simulink model "ACTIVITY_01_DR_CHAIREZ"  (R2022a)
settings: Solver=VariableStepAuto  StartTime=0.0  StopTime=1  RelTol=1e-3
libraries: slpidlib x2
settings Model: Creator=Pitip  LastModifiedBy=Pitip

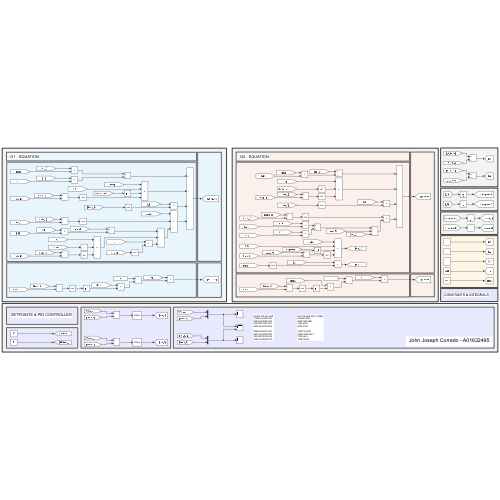
[thumbnail: Simulink's stored preview of the top-level diagram]
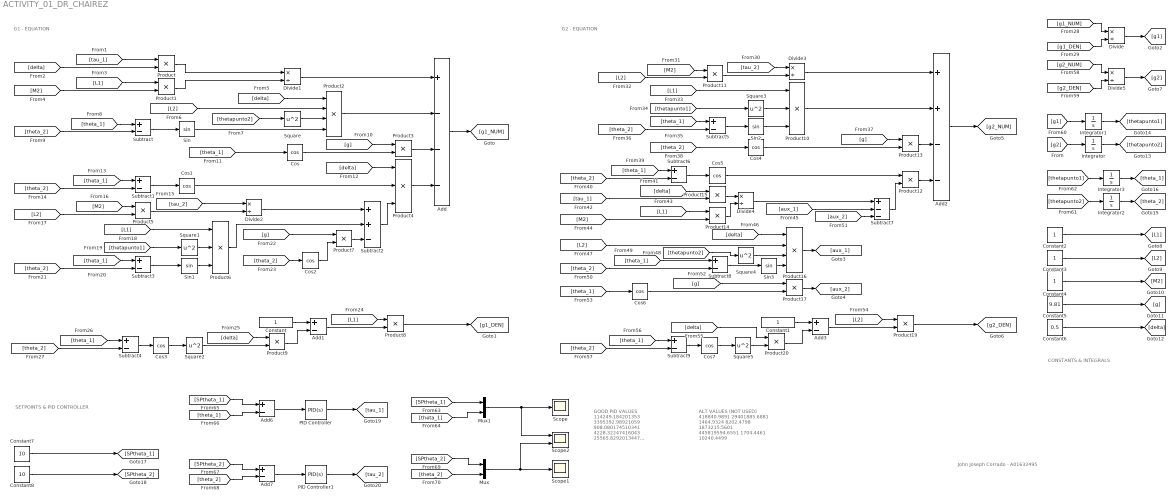
== system ACTIVITY_01_DR_CHAIREZ ==
  note: G1 - EQUATION
  note: ALT VALUES (NOT USED)
      | 418840.9891
      | 29401885.6881
      | 1464.9324
      | 8202.4798
      |
      | 1873215.5601
      | 445819594.6551
      | 1704.4461
      | 10240.4499
  note: SETPOINTS & PID CONTROLLER
  note: John Joseph Corrado - A01632495
  note: GOOD PID VALUES
      | 114249.184201353
      | 3395392.98921059
      | 908.080174510341
      | 4228.32247416043
      |
      | 25565.8292013447
      | 389143.824057423
      | 335.250158154316
      | 34347.6360627222
  note: G2 - EQUATION
  note: CONSTANTS & INTEGRALS
  Add : Sum  Inputs=+---
  Add{1,3,6..7} (4 alike) : Sum  Inputs=+-
  Add2 : Sum  Inputs=++--
  Constant{,1..4} (5 alike) : Constant
  Constant5 : Constant  Value=9.81
  Constant6 : Constant  Value=0.5
  Constant7 : Constant  Value=10
  Constant8 : Constant  Value=10
  Cos{,1..7} (8 alike) : Trigonometry  Operator=cos
  Divide{,1..5} (6 alike) : Product  Inputs=*/
  Integrator{,1..3} (4 alike) : Integrator
  Mux : Mux  Inputs=2
  Mux1 : Mux  Inputs=2
  PID Controller : slpidlib/PID Controller  Controller=PID  Form=Parallel  TimeDomain=Continuous-time  UseExternalTs=off  SampleTime=-1  IntegratorMethod=Forward Euler  FilterMethod=Forward Euler  ControllerParametersSource=internal  P=114249.184201353  I=3395392.98921059  UseKiTs=off  D=908.080174510341  N=4228.32247416043  UseFilter=on  TunerSelectOption=Transfer Function Based (PID Tuner App)  InitialConditionSource=internal  InitialConditionForIntegrator=0  InitialConditionForFilter=0  DifferentiatorICPrevScaledInput=0  ExternalReset=none  TrackingMode=off  Kt=1  LimitOutput=off  SatLimitsSource=internal  UpperSaturationLimit=inf  LowerSaturationLimit=-inf  LinearizeAsGain=on  AntiWindupMode=none  Kb=1  POutMin=[]  POutMax=[]  IOutMin=[]  IOutMax=[]  DOutMin=[]  DOutMax=[]  NOutMin=[]  NOutMax=[]  SumOutMin=[]  SumOutMax=[]  SaturationOutMin=[]  SaturationOutMax=[]  PParamMin=[]  PParamMax=[]  IParamMin=[]  IParamMax=[]  DParamMin=[]  DParamMax=[]  NParamMin=[]  NParamMax=[]  KbParamMin=[]  KbParamMax=[]  KtParamMin=[]  KtParamMax=[]  KbOutMin=[]  KbOutMax=[]  KtOutMin=[]  KtOutMax=[]  IntegratorOutMin=[]  IntegratorOutMax=[]  FilterOutMin=[]  FilterOutMax=[]  SumI1OutMin=[]  SumI1OutMax=[]  SumI2OutMin=[]  SumI2OutMax=[]  SumI3OutMin=[]  SumI3OutMax=[]  SumI4OutMin=[]  SumI4OutMax=[]  SumDOutMin=[]  SumDOutMax=[]  DifferentiatorOutMin=[]  DifferentiatorOutMax=[]  FilterDiffOutCoefMin=[]  FilterDiffOutCoefMax=[]  ReciprocalOutMin=[]  ReciprocalOutMax=[]  SumDenOutMin=[]  SumDenOutMax=[]  SumNumOutMin=[]  SumNumOutMax=[]  DivideOutMin=[]  DivideOutMax=[]  UdiffTsProdOutMin=[]  UdiffTsProdOutMax=[]  NTsProdOutMin=[]  NTsProdOutMax=[]  UintegralTsProdOutMin=[]  UintegralTsProdOutMax=[]  UngainTsProdOutMin=[]  UngainTsProdOutMax=[]  IntegratorContinuousStateAttributes=''  IntegratorStateMustResolveToSignalObject=off  IntegratorRTWStateStorageClass=Auto  FilterContinuousStateAttributes=''  FilterStateMustResolveToSignalObject=off  FilterRTWStateStorageClass=Auto  ParallelPVariant=InternalParameters  IdealPVariant=Disabled  IVariant=InternalParameters  DVariant=InternalParameters  IntegratorVariant=Continuous  SatVariant=Disabled  AWVariant=Passthrough  PCopyVariant=Disabled  TRVariant=Disabled  FdbkBlocksVariant=Forward  IdealPFdbkVariant=Disabled  SatFdbkVariant=Disabled  DerivativeFilterVariant=ContFilter  NVariant=InternalParameters  NCopyVariant=Disabled  FilterICVariant=InternalICsFilter  IntegratorICVariant=InternalICs  ExternalResetVariant=Disabled  TRSumVariant=Passthrough  SumFdbkVariant=Disabled  SumVariant=Sum_PID  TsampFilterVariant=InternalTs  TsampNgainVariant=Passthrough  TsampIntegralVariant=Passthrough  ExternalSaturationOutDataTypeStr=Inherit: Same as second input  aMode=0
  PID Controller1 : slpidlib/PID Controller  Controller=PID  Form=Parallel  TimeDomain=Continuous-time  UseExternalTs=off  SampleTime=-1  IntegratorMethod=Forward Euler  FilterMethod=Forward Euler  ControllerParametersSource=internal  P=25565.8292013447  I=389143.824057423  UseKiTs=off  D=335.250158154316  N=34347.6360627222  UseFilter=on  TunerSelectOption=Transfer Function Based (PID Tuner App)  InitialConditionSource=internal  InitialConditionForIntegrator=0  InitialConditionForFilter=0  DifferentiatorICPrevScaledInput=0  ExternalReset=none  TrackingMode=off  Kt=1  LimitOutput=off  SatLimitsSource=internal  UpperSaturationLimit=inf  LowerSaturationLimit=-inf  LinearizeAsGain=on  AntiWindupMode=none  Kb=1  POutMin=[]  POutMax=[]  IOutMin=[]  IOutMax=[]  DOutMin=[]  DOutMax=[]  NOutMin=[]  NOutMax=[]  SumOutMin=[]  SumOutMax=[]  SaturationOutMin=[]  SaturationOutMax=[]  PParamMin=[]  PParamMax=[]  IParamMin=[]  IParamMax=[]  DParamMin=[]  DParamMax=[]  NParamMin=[]  NParamMax=[]  KbParamMin=[]  KbParamMax=[]  KtParamMin=[]  KtParamMax=[]  KbOutMin=[]  KbOutMax=[]  KtOutMin=[]  KtOutMax=[]  IntegratorOutMin=[]  IntegratorOutMax=[]  FilterOutMin=[]  FilterOutMax=[]  SumI1OutMin=[]  SumI1OutMax=[]  SumI2OutMin=[]  SumI2OutMax=[]  SumI3OutMin=[]  SumI3OutMax=[]  SumI4OutMin=[]  SumI4OutMax=[]  SumDOutMin=[]  SumDOutMax=[]  DifferentiatorOutMin=[]  DifferentiatorOutMax=[]  FilterDiffOutCoefMin=[]  FilterDiffOutCoefMax=[]  ReciprocalOutMin=[]  ReciprocalOutMax=[]  SumDenOutMin=[]  SumDenOutMax=[]  SumNumOutMin=[]  SumNumOutMax=[]  DivideOutMin=[]  DivideOutMax=[]  UdiffTsProdOutMin=[]  UdiffTsProdOutMax=[]  NTsProdOutMin=[]  NTsProdOutMax=[]  UintegralTsProdOutMin=[]  UintegralTsProdOutMax=[]  UngainTsProdOutMin=[]  UngainTsProdOutMax=[]  IntegratorContinuousStateAttributes=''  IntegratorStateMustResolveToSignalObject=off  IntegratorRTWStateStorageClass=Auto  FilterContinuousStateAttributes=''  FilterStateMustResolveToSignalObject=off  FilterRTWStateStorageClass=Auto  ParallelPVariant=InternalParameters  IdealPVariant=Disabled  IVariant=InternalParameters  DVariant=InternalParameters  IntegratorVariant=Continuous  SatVariant=Disabled  AWVariant=Passthrough  PCopyVariant=Disabled  TRVariant=Disabled  FdbkBlocksVariant=Forward  IdealPFdbkVariant=Disabled  SatFdbkVariant=Disabled  DerivativeFilterVariant=ContFilter  NVariant=InternalParameters  NCopyVariant=Disabled  FilterICVariant=InternalICsFilter  IntegratorICVariant=InternalICs  ExternalResetVariant=Disabled  TRSumVariant=Passthrough  SumFdbkVariant=Disabled  SumVariant=Sum_PID  TsampFilterVariant=InternalTs  TsampNgainVariant=Passthrough  TsampIntegralVariant=Passthrough  ExternalSaturationOutDataTypeStr=Inherit: Same as second input  aMode=0
  Product{,1,3,5,7..9,11..15,17,19..20} (15 alike) : Product
  Product10 : Product  Inputs=3
  Product16 : Product  Inputs=4
  Product2 : Product  Inputs=4
  Product4 : Product  Inputs=3
  Product6 : Product  Inputs=3
  Scope : Scope
  Scope1 : Scope
  Scope2 : Scope  NumInputPorts=2
  Sin{,1..3} (4 alike) : Trigonometry
  Square{,1..5} (6 alike) : Math  Operator=square
  Subtract{,1,3..6,8..9} (8 alike) : Sum  Inputs=+-
  Subtract2 : Sum  Inputs=++-
  Subtract7 : Sum  Inputs=+--
  wires:
  Divide1/1 -> Add/1
  Product/1 -> Divide1/1
  Product1/1 -> Divide1/2
  [tau_1] -> Product/1
  [delta] -> Product/2
  [L1] -> Product1/1
  [M2] -> Product1/2
  [delta] -> Product2/1
  Product2/1 -> Add/2
  [L2] -> Product2/2
  Square/1 -> Product2/3
  [thetapunto2] -> Square/1
  Sin/1 -> Product2/4
  Subtract/1 -> Sin/1
  [theta_1] -> Subtract/1
  [theta_2] -> Subtract/2
  Product3/1 -> Add/3
  [g] -> Product3/1
  Cos/1 -> Product3/2
  [theta_1] -> Cos/1
  [delta] -> Product4/1
  Product4/1 -> Add/4
  Cos1/1 -> Product4/2
  [theta_2] -> Subtract1/2
  [theta_1] -> Subtract1/1
  Subtract1/1 -> Cos1/1
  Subtract2/1 -> Product4/3
  [tau_2] -> Divide2/1
  Product5/1 -> Divide2/2
  [M2] -> Product5/1
  [L2] -> Product5/2
  Divide2/1 -> Subtract2/1
  Product6/1 -> Subtract2/2
  [L1] -> Product6/1
  Square1/1 -> Product6/2
  [thetapunto1] -> Square1/1
  [theta_2] -> Subtract3/2
  Subtract3/1 -> Sin1/1
  [theta_1] -> Subtract3/1
  Sin1/1 -> Product6/3
  Product7/1 -> Subtract2/3
  [g] -> Product7/1
  [theta_2] -> Cos2/1
  Cos2/1 -> Product7/2
  Add/1 -> [g1_NUM]
  Add1/1 -> Product8/2
  [L1] -> Product8/1
  Constant/1 -> Add1/1
  Product9/1 -> Add1/2
  [delta] -> Product9/1
  Subtract4/1 -> Cos3/1
  [theta_1] -> Subtract4/1
  [theta_2] -> Subtract4/2
  Square2/1 -> Product9/2
  Cos3/1 -> Square2/1
  Product8/1 -> [g1_DEN]
  [g1_NUM] -> Divide/1
  [g1_DEN] -> Divide/2
  Divide/1 -> [g1]
  Divide3/1 -> Add2/1
  [tau_2] -> Divide3/1
  Product11/1 -> Divide3/2
  [L2] -> Product11/2
  [M2] -> Product11/1
  Product10/1 -> Add2/2
  [L1] -> Product10/1
  Square3/1 -> Product10/2
  [thetapunto1] -> Square3/1
  Sin2/1 -> Product10/3
  [theta_2] -> Subtract5/2
  [theta_1] -> Subtract5/1
  Subtract5/1 -> Sin2/1
  [theta_2] -> Cos4/1
  Cos4/1 -> Product13/2
  [g] -> Product13/1
  Product13/1 -> Add2/3
  Product12/1 -> Add2/4
  [theta_2] -> Subtract6/2
  Subtract6/1 -> Cos5/1
  [theta_1] -> Subtract6/1
  Cos5/1 -> Product12/1
  Subtract7/1 -> Product12/2
  Divide4/1 -> Subtract7/1
  [L1] -> Product14/1
  [M2] -> Product14/2
  Product15/1 -> Divide4/1
  [delta] -> Product15/1
  [tau_1] -> Product15/2
  Product14/1 -> Divide4/2
  [aux_1] -> Subtract7/2
  Product16/1 -> [aux_1]
  [delta] -> Product16/1
  [L2] -> Product16/2
  [thetapunto2] -> Square4/1
  Square4/1 -> Product16/3
  [theta_2] -> Subtract8/2
  [theta_1] -> Subtract8/1
  Subtract8/1 -> Sin3/1
  Sin3/1 -> Product16/4
  [aux_2] -> Subtract7/3
  Product17/1 -> [aux_2]
  [g] -> Product17/1
  [theta_1] -> Cos6/1
  Cos6/1 -> Product17/2
  Add2/1 -> [g2_NUM]
  Add3/1 -> Product19/2
  [theta_2] -> Subtract9/2
  [theta_1] -> Subtract9/1
  Subtract9/1 -> Cos7/1
  Product20/1 -> Add3/2
  Cos7/1 -> Square5/1
  [L2] -> Product19/1
  Constant1/1 -> Add3/1
  [delta] -> Product20/1
  Square5/1 -> Product20/2
  Product19/1 -> [g2_DEN]
  [g2_NUM] -> Divide5/1
  Divide5/1 -> [g2]
  [g2_DEN] -> Divide5/2
  Constant2/1 -> [L1]
  Constant3/1 -> [L2]
  Constant5/1 -> [g]
  Constant4/1 -> [M2]
  Constant6/1 -> [delta]
  [g2] -> Integrator/1
  Integrator/1 -> [thetapunto2]
  [g1] -> Integrator1/1
  Integrator1/1 -> [thetapunto1]
  Integrator3/1 -> [theta_1]
  [thetapunto2] -> Integrator2/1
  [thetapunto1] -> Integrator3/1
  Integrator2/1 -> [theta_2]
  [theta_1] -> Add6/2
  [SPtheta_1] -> Add6/1
  [theta_2] -> Add7/2
  [SPtheta_2] -> Add7/1
  Add6/1 -> PID Controller/1
  Add7/1 -> PID Controller1/1
  PID Controller/1 -> [tau_1]
  PID Controller1/1 -> [tau_2]
  Constant7/1 -> [SPtheta_1]
  Constant8/1 -> [SPtheta_2]
  [SPtheta_2] -> Mux/1
  [theta_2] -> Mux/2
  [SPtheta_1] -> Mux1/1
  [theta_1] -> Mux1/2
  Mux1/1 -> Scope2/1, Scope/1
  Mux/1 -> Scope2/2, Scope1/1
